simulink model "current_loop"  (R2020a)
settings: Solver=VariableStepAuto  StartTime=0.0  StopTime=Tsim  MaxStep=Ts/10  RelTol=1e-3
values from neighbouring files (symbols this model uses):
  we = 2*pi*50    (= 314.159265359)    [init.m]
libraries: powerlib_meascontrol x2
settings Model: Creator=Ivan  LastModifiedBy=Ivan

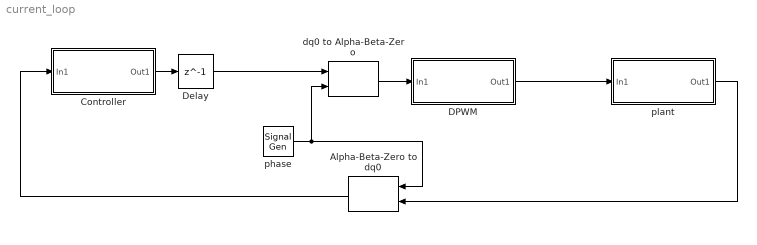
== system current_loop ==
  Alpha-Beta-Zero to dq0 : powerlib_meascontrol/Transformations/Alpha-Beta-Zero to dq0  Alignment=90 degrees behind phase A axis
  Controller : Subsystem
  DPWM : Subsystem
  Delay : Delay  DelayLength=1  InitialCondition=0
  dq0 to Alpha-Beta-Zero : powerlib_meascontrol/Transformations/dq0 to Alpha-Beta-Zero  Alignment=90 degrees behind phase A axis
      settings: SourceProductBaseCode=PS
  phase : SignalGenerator  WaveForm=sawtooth  Amplitude=2*pi  Frequency=we  Units=rad/sec
  plant : Subsystem
  wires:
  Controller/1(Out1) -> Delay/1
  Delay/1 -> dq0 to Alpha-Beta-Zero/1
  dq0 to Alpha-Beta-Zero/1 -> DPWM/1(In1)
  DPWM/1(Out1) -> plant/1(In1)
  plant/1(Out1) -> Alpha-Beta-Zero to dq0/1
  phase/1 -> Alpha-Beta-Zero to dq0/2, dq0 to Alpha-Beta-Zero/2
  Alpha-Beta-Zero to dq0/1 -> Controller/1(In1)

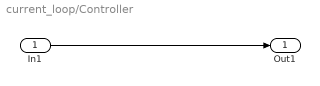
== system current_loop/Controller ==
  In1 : Inport
  Out1 : Outport
  wires:
  In1/1 -> Out1/1

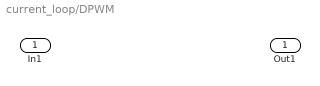
== system current_loop/DPWM ==
  In1 : Inport
  Out1 : Outport

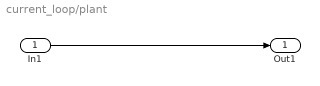
== system current_loop/plant ==
  In1 : Inport
  Out1 : Outport
  wires:
  In1/1 -> Out1/1
